simulink model "threeDOFSim"  (R2024b)
settings: Solver=VariableStepAuto  StartTime=0.0  StopTime=7.13  RelTol=1e-3
settings Model: Creator=rog  LastModifiedBy=noahbliss
settings DebuggingCC: AlgebraicLoopMsg=none

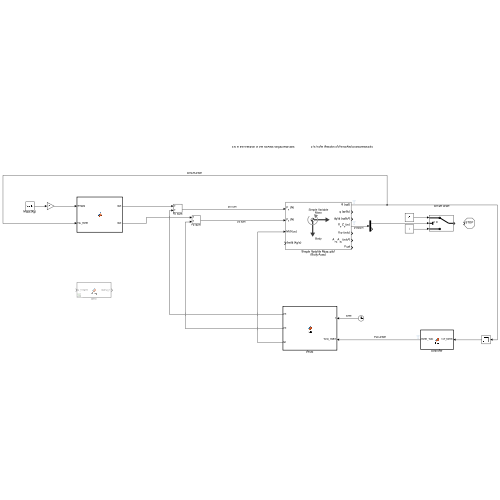
[thumbnail: Simulink's stored preview of the top-level diagram]
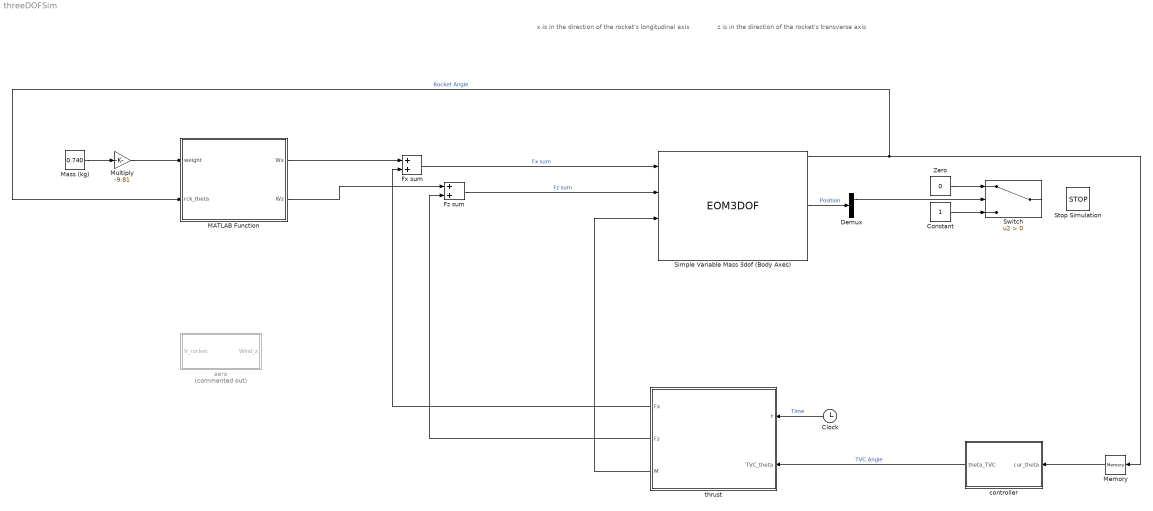
== system threeDOFSim ==
  note: z is in the direction of the rocket's transverse axis
  note: x is in the direction of the rocket's longitudinal axis
  Clock : Clock
  Constant : Constant
  Demux : Demux  Outputs=2
  Fx sum : Sum
  Fz sum : Sum
  MATLAB Function : MATLAB Function  TreatAsAtomicUnit=on
  Mass (kg) : Constant  Value=0.740
  Memory : Memory
  Multiply : Gain  Gain=-9.81
  Simple Variable Mass 3dof (Body Axes) : EOM3DOF  mtype=Simple Variable  v_ini=0  theta_ini=0.1  pos_ini=[0.01 0]  mass=0.740  mass_e=0.690  mass_f=0.740  Iyy_e=3.10  Iyy_f=3.22  g=0
  Stop Simulation : Stop
  Switch : Switch  Criteria=u2 > Threshold  SaturateOnIntegerOverflow=off  InputSameDT=off
  Zero : Constant  Value=0  OutDataTypeStr=Inherit: Inherit via back propagation
  aero : MATLAB Function  Commented=on  TreatAsAtomicUnit=on
  controller : MATLAB Function  TreatAsAtomicUnit=on
  thrust : MATLAB Function  TreatAsAtomicUnit=on
  wires:
  Clock/1 -> thrust/1(t)  "Time"
  thrust/3(M) -> Simple Variable Mass 3dof (Body Axes)/3
  thrust/1(Fx) -> Fx sum/2
  Fx sum/1 -> Simple Variable Mass 3dof (Body Axes)/1  "Fx sum"
  Simple Variable Mass 3dof (Body Axes)/1 -> Memory/1, MATLAB Function/2(rck_theta)  "Rocket Angle"
  Mass (kg)/1 -> Multiply/1
  thrust/2(Fz) -> Fz sum/2
  Fz sum/1 -> Simple Variable Mass 3dof (Body Axes)/2  "Fz sum"
  controller/1(theta_TVC) -> thrust/2(TVC_theta)  "TVC Angle"
  Simple Variable Mass 3dof (Body Axes)/4 -> Demux/1  "Position"
  Memory/1 -> controller/1(cur_theta)
  Constant/1 -> Switch/3
  Zero/1 -> Switch/1
  Demux/1 -> Switch/2
  Multiply/1 -> MATLAB Function/1(weight)
  MATLAB Function/1(Wx) -> Fx sum/1
  MATLAB Function/2(Wz) -> Fz sum/1

== matlab function threeDOFSim/controller ==
  data: cur_theta input; theta_TVC output
function theta_TVC = fcn(cur_theta)   
   % constants
    theta_desired = 0;  
    Kp = 15;  
    Ki = 0.35;    
    Kd = 0.05;
    filter_tau = 1; 
    max_TVC_angle=deg2rad(7.5);

    persistent integral_error prev_error prev_d;

    if isempty(integral_error)
        integral_error = 0;
        prev_error = 0;
        prev_d = 0;
    end

 


    current_error = theta_desired - cur_theta;

    integral_error = integral_error + current_error; % add back integral_error*leaky_control

    % Derivative Term (Filtered)
    derivative_error = (current_error - prev_error);
    filtered_d = (filter_tau * prev_d + derivative_error) / (filter_tau + 1);
    
    % Compute PID Output
    theta_TVC = (Kp * current_error + Ki * integral_error + Kd * filtered_d);
    

    % Update Previous Values
    prev_error = current_error;
    prev_d = filtered_d;

    if theta_TVC>max_TVC_angle
        theta_TVC=max_TVC_angle;
    elseif theta_TVC<-max_TVC_angle
        theta_TVC=-max_TVC_angle;
    end

end

== matlab function threeDOFSim/thrust ==
  data: t input; Fx output; TVC_theta input; Fz output; M output
function [Fx, Fz, M] = fcn(t, TVC_theta)

    persistent loadedData;
    
    %pitch is TVC angle
    %rck_theta is rocket angle

    if isempty(loadedData)
        loadedData = load('F10ThrustCurve.mat');
    end

    thrust_interp = interp1(loadedData.F10ThrustCurve(:,1), loadedData.F10ThrustCurve(:,2), t);

    burnout_time = 7.13;
    if t < burnout_time
        T = thrust_interp;
    else
        T = 0;
    end

    
    % Compute forces due to thrust
    Fx = T * cos(TVC_theta);
    Fz = T * sin(TVC_theta);

    COM_distance = 0.23;
    M = COM_distance*(T*sin(TVC_theta));
end

== matlab function threeDOFSim/aero ==
  data: V_rocket input; Wind_z output
function Wind_z = drag(V_rocket)
    rho = 1;    
    C_D = 0.75;   
    A = 1.5;      

    %Drag coef=0.47

    %Wind
    V_wind_z = normrnd(0, 3);  
    
    V_eff_z = V_rocket - V_wind_z;
    V_eff = abs(V_eff_x);
    
    F_drag = 0.5 * rho * V_eff^2 * C_D * A;
    
    Wind_z = F_drag * (V_eff / V_eff_z); 
end

== matlab function threeDOFSim/MATLAB Function ==
  data: weight input; Wx output; rck_theta input; Wz output
function [Wx,Wz] = fcn(weight,rck_theta)

Wx=weight*cos(rck_theta);
Wz=weight*sin(rck_theta);
